simulink model "ACR_4_Saturation_5"  (R2020a)
settings: Solver=ode45  StartTime=0.0  StopTime=10.0  MaxStep=1e-5  RelTol=1e-3
libraries: simulink x1
settings Model: Creator=78253  LastModifiedBy=78253

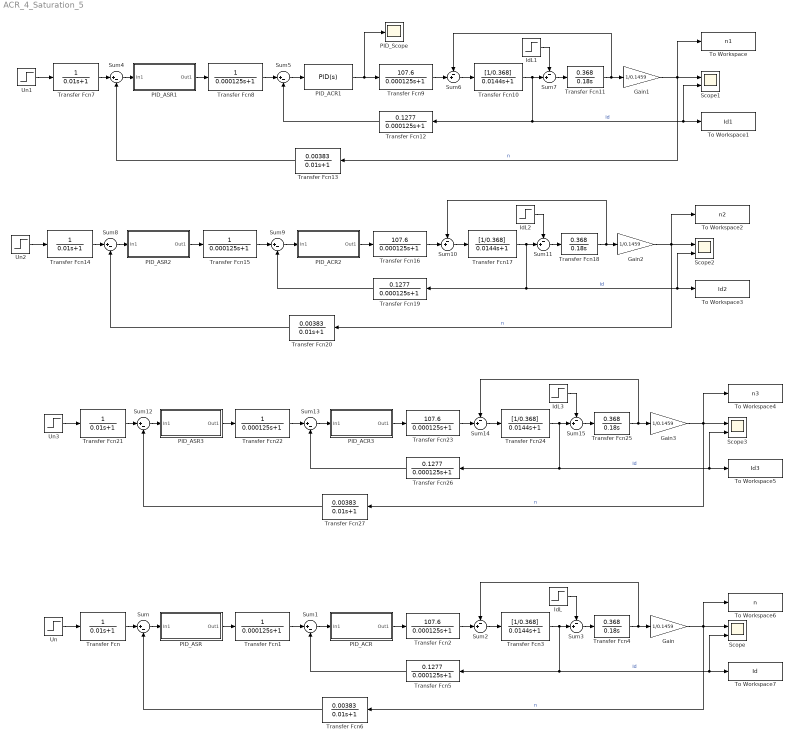
== system ACR_4_Saturation_5 ==
  Gain{,1..3} (4 alike) : Gain  Gain=1/0.1459
  IdL{,1..3} (4 alike) : Step  Time=0  After=52.2  SampleTime=0
  PID_ACR : Subsystem
  PID_ACR1 : simulink/Continuous/PID Controller  Controller=PID  Form=Parallel  TimeDomain=Continuous-time  UseExternalTs=off  SampleTime=-1  IntegratorMethod=Forward Euler  FilterMethod=Forward Euler  ControllerParametersSource=internal  P=0.771  I=53.542  D=0  UseFilter=on  N=100  TunerSelectOption=Transfer Function Based (PID Tuner App)  InitialConditionSource=internal  InitialConditionForIntegrator=0  InitialConditionForFilter=0  DifferentiatorICPrevScaledInput=0  ExternalReset=none  TrackingMode=off  Kt=1  LimitOutput=on  UpperSaturationLimit=5  LowerSaturationLimit=-5  LinearizeAsGain=on  AntiWindupMode=none  Kb=1  POutMin=[]  POutMax=[]  IOutMin=[]  IOutMax=[]  DOutMin=[]  DOutMax=[]  NOutMin=[]  NOutMax=[]  SumOutMin=[]  SumOutMax=[]  SaturationOutMin=[]  SaturationOutMax=[]  PParamMin=[]  PParamMax=[]  IParamMin=[]  IParamMax=[]  DParamMin=[]  DParamMax=[]  NParamMin=[]  NParamMax=[]  KbParamMin=[]  KbParamMax=[]  KtParamMin=[]  KtParamMax=[]  KbOutMin=[]  KbOutMax=[]  KtOutMin=[]  KtOutMax=[]  IntegratorOutMin=[]  IntegratorOutMax=[]  FilterOutMin=[]  FilterOutMax=[]  SumI1OutMin=[]  SumI1OutMax=[]  SumI2OutMin=[]  SumI2OutMax=[]  SumI3OutMin=[]  SumI3OutMax=[]  SumI4OutMin=[]  SumI4OutMax=[]  SumDOutMin=[]  SumDOutMax=[]  DifferentiatorOutMin=[]  DifferentiatorOutMax=[]  FilterDiffOutCoefMin=[]  FilterDiffOutCoefMax=[]  ReciprocalOutMin=[]  ReciprocalOutMax=[]  SumDenOutMin=[]  SumDenOutMax=[]  SumNumOutMin=[]  SumNumOutMax=[]  DivideOutMin=[]  DivideOutMax=[]  UdiffTsProdOutMin=[]  UdiffTsProdOutMax=[]  NTsProdOutMin=[]  NTsProdOutMax=[]  UintegralTsProdOutMin=[]  UintegralTsProdOutMax=[]  UngainTsProdOutMin=[]  UngainTsProdOutMax=[]  IntegratorContinuousStateAttributes=''  IntegratorStateMustResolveToSignalObject=off  IntegratorRTWStateStorageClass=Auto  FilterContinuousStateAttributes=''  FilterStateMustResolveToSignalObject=off  FilterRTWStateStorageClass=Auto  ParallelPVariant=InternalParameters  IdealPVariant=Disabled  IVariant=InternalParameters  DVariant=InternalParameters  IntegratorVariant=Continuous  SatVariant=Enabled  AWVariant=Passthrough  PCopyVariant=Disabled  TRVariant=Disabled  FdbkBlocksVariant=Forward  IdealPFdbkVariant=Disabled  SatFdbkVariant=Disabled  DerivativeFilterVariant=ContFilter  NVariant=InternalParameters  NCopyVariant=Disabled  FilterICVariant=InternalICsFilter  IntegratorICVariant=InternalICs  ExternalResetVariant=Disabled  TRSumVariant=Passthrough  SumFdbkVariant=Disabled  SumVariant=Sum_PID  TsampFilterVariant=InternalTs  TsampNgainVariant=Passthrough  TsampIntegralVariant=Passthrough
  PID_ACR2 : Subsystem
  PID_ACR3 : Subsystem
  PID_ASR : Subsystem
  PID_ASR1 : Subsystem
  PID_ASR2 : Subsystem
  PID_ASR3 : Subsystem
  PID_Scope : Scope
  Scope{,1..3} (4 alike) : Scope  NumInputPorts=2
  Sum{,1,4..5,8..9,12..13} (8 alike) : Sum  Inputs=|+-
  Sum{2..3,6..7,10..11,14..15} (8 alike) : Sum  Inputs=-+|
  To Workspace : ToWorkspace  VariableName=n1  SaveFormat=Timeseries  SampleTime=-1
  To Workspace1 : ToWorkspace  VariableName=Id1  SaveFormat=Timeseries  SampleTime=-1
  To Workspace2 : ToWorkspace  VariableName=n2  SaveFormat=Timeseries  SampleTime=-1
  To Workspace3 : ToWorkspace  VariableName=Id2  SaveFormat=Timeseries  SampleTime=-1
  To Workspace4 : ToWorkspace  VariableName=n3  SaveFormat=Timeseries  SampleTime=-1
  To Workspace5 : ToWorkspace  VariableName=Id3  SaveFormat=Timeseries  SampleTime=-1
  To Workspace6 : ToWorkspace  VariableName=n  SaveFormat=Timeseries  SampleTime=-1
  To Workspace7 : ToWorkspace  VariableName=Id  SaveFormat=Timeseries  SampleTime=-1
  Transfer Fcn{,7,14,21} (4 alike) : TransferFcn  Denominator=[0.01 1]
  Transfer Fcn{1,8,15,22} (4 alike) : TransferFcn  Denominator=[0.000125 1]
  Transfer Fcn{3,10,17,24} (4 alike) : TransferFcn  Numerator=[1/0.368]  Denominator=[0.0144 1]
  Transfer Fcn{4,11,18,25} (4 alike) : TransferFcn  Numerator=[0.368]  Denominator=[0.18 0]
  Transfer Fcn{5,12,19,26} (4 alike) : TransferFcn  Numerator=[0.1277]  Denominator=[0.000125 1]
  Transfer Fcn{6,13,20,27} (4 alike) : TransferFcn  Numerator=[0.00383]  Denominator=[0.01 1]
  Transfer Fcn{2,9,16,23} (4 alike) : TransferFcn  Numerator=[107.6]  Denominator=[0.000125 1]
  Un{,1..3} (4 alike) : Step  Time=0  After=10  SampleTime=0
  wires:
  Sum3/1 -> Transfer Fcn4/1
  Transfer Fcn/1 -> Sum/1
  Sum2/1 -> Transfer Fcn3/1
  Un/1 -> Transfer Fcn/1
  Transfer Fcn5/1 -> Sum1/2
  Transfer Fcn6/1 -> Sum/2
  PID_ACR/1(Out1) -> Transfer Fcn2/1
  Transfer Fcn1/1 -> Sum1/1
  IdL/1 -> Sum3/1
  Transfer Fcn4/1 -> Sum2/1, Gain/1
  Transfer Fcn3/1 -> Transfer Fcn5/1, Scope/2, To Workspace7/1, Sum3/2  "Id"
  Gain/1 -> To Workspace6/1, Transfer Fcn6/1, Scope/1  "n"
  Sum/1 -> PID_ASR/1(In1)
  Sum1/1 -> PID_ACR/1(In1)
  Transfer Fcn2/1 -> Sum2/2
  PID_ASR/1(Out1) -> Transfer Fcn1/1
  PID_ASR1/1(Out1) -> Transfer Fcn8/1
  Transfer Fcn10/1 -> Transfer Fcn12/1, Scope1/2, To Workspace1/1, Sum7/2  "Id"
  Transfer Fcn9/1 -> Sum6/2
  Gain1/1 -> To Workspace/1, Transfer Fcn13/1, Scope1/1  "n"
  Transfer Fcn8/1 -> Sum5/1
  Transfer Fcn13/1 -> Sum4/2
  Sum4/1 -> PID_ASR1/1(In1)
  IdL1/1 -> Sum7/1
  Transfer Fcn7/1 -> Sum4/1
  Transfer Fcn12/1 -> Sum5/2
  Un1/1 -> Transfer Fcn7/1
  Sum6/1 -> Transfer Fcn10/1
  Transfer Fcn11/1 -> Sum6/1, Gain1/1
  Sum7/1 -> Transfer Fcn11/1
  PID_ASR2/1(Out1) -> Transfer Fcn15/1
  Transfer Fcn17/1 -> Transfer Fcn19/1, To Workspace3/1, Scope2/2, Sum11/2  "Id"
  Transfer Fcn16/1 -> Sum10/2
  Gain2/1 -> To Workspace2/1, Transfer Fcn20/1, Scope2/1  "n"
  Sum9/1 -> PID_ACR2/1(In1)
  Transfer Fcn15/1 -> Sum9/1
  Transfer Fcn20/1 -> Sum8/2
  PID_ACR2/1(Out1) -> Transfer Fcn16/1
  Sum8/1 -> PID_ASR2/1(In1)
  IdL2/1 -> Sum11/1
  Transfer Fcn14/1 -> Sum8/1
  Transfer Fcn19/1 -> Sum9/2
  Un2/1 -> Transfer Fcn14/1
  Sum10/1 -> Transfer Fcn17/1
  Transfer Fcn18/1 -> Sum10/1, Gain2/1
  Sum11/1 -> Transfer Fcn18/1
  PID_ASR3/1(Out1) -> Transfer Fcn22/1
  Transfer Fcn24/1 -> Transfer Fcn26/1, To Workspace5/1, Scope3/2, Sum15/2  "Id"
  Transfer Fcn23/1 -> Sum14/2
  Gain3/1 -> To Workspace4/1, Transfer Fcn27/1, Scope3/1  "n"
  Sum13/1 -> PID_ACR3/1(In1)
  Transfer Fcn22/1 -> Sum13/1
  Transfer Fcn27/1 -> Sum12/2
  PID_ACR3/1(Out1) -> Transfer Fcn23/1
  Sum12/1 -> PID_ASR3/1(In1)
  IdL3/1 -> Sum15/1
  Transfer Fcn21/1 -> Sum12/1
  Transfer Fcn26/1 -> Sum13/2
  Un3/1 -> Transfer Fcn21/1
  Sum14/1 -> Transfer Fcn24/1
  Transfer Fcn25/1 -> Sum14/1, Gain3/1
  Sum15/1 -> Transfer Fcn25/1
  PID_ACR1/1 -> PID_Scope/1, Transfer Fcn9/1
  Sum5/1 -> PID_ACR1/1

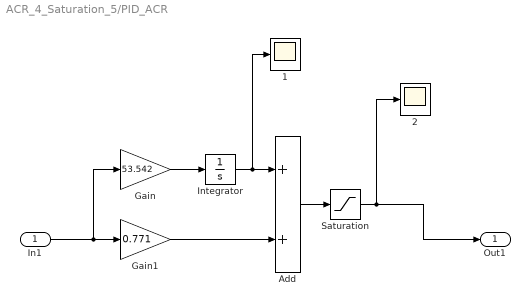
== system ACR_4_Saturation_5/PID_ACR ==
  In1 : Inport
  1 : Scope
  2 : Scope
  Add : Sum
  Gain : Gain  Gain=53.542
  Gain1 : Gain  Gain=0.771
  Integrator : Integrator  LimitOutput=on  UpperSaturationLimit=5  LowerSaturationLimit=-5
  Saturation : Saturate  UpperLimit=5  LowerLimit=-5
  Out1 : Outport
  wires:
  In1/1 -> Gain/1, Gain1/1
  Gain1/1 -> Add/2
  Add/1 -> Saturation/1
  Gain/1 -> Integrator/1
  Saturation/1 -> Out1/1, 2/1
  Integrator/1 -> 1/1, Add/1

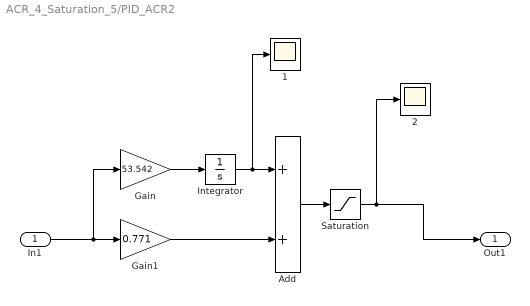
== system ACR_4_Saturation_5/PID_ACR2 ==
  In1 : Inport
  1 : Scope
  2 : Scope
  Add : Sum
  Gain : Gain  Gain=53.542
  Gain1 : Gain  Gain=0.771
  Integrator : Integrator  UpperSaturationLimit=5  LowerSaturationLimit=-5
  Saturation : Saturate  UpperLimit=5  LowerLimit=-5
  Out1 : Outport
  wires:
  In1/1 -> Gain/1, Gain1/1
  Gain1/1 -> Add/2
  Add/1 -> Saturation/1
  Gain/1 -> Integrator/1
  Saturation/1 -> Out1/1, 2/1
  Integrator/1 -> 1/1, Add/1

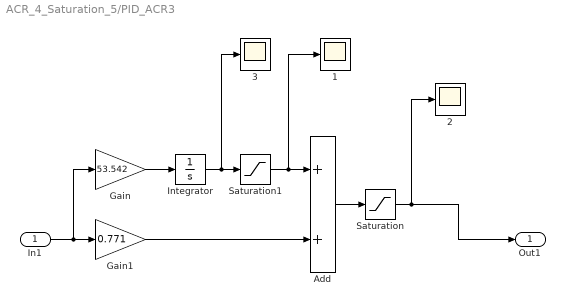
== system ACR_4_Saturation_5/PID_ACR3 ==
  In1 : Inport
  1 : Scope
  2 : Scope
  3 : Scope
  Add : Sum
  Gain : Gain  Gain=53.542
  Gain1 : Gain  Gain=0.771
  Integrator : Integrator  UpperSaturationLimit=5  LowerSaturationLimit=-5
  Saturation : Saturate  UpperLimit=5  LowerLimit=-5
  Saturation1 : Saturate  UpperLimit=5  LowerLimit=-5
  Out1 : Outport
  wires:
  In1/1 -> Gain1/1, Gain/1
  Gain1/1 -> Add/2
  Add/1 -> Saturation/1
  Gain/1 -> Integrator/1
  Saturation/1 -> Out1/1, 2/1
  Integrator/1 -> 3/1, Saturation1/1
  Saturation1/1 -> 1/1, Add/1

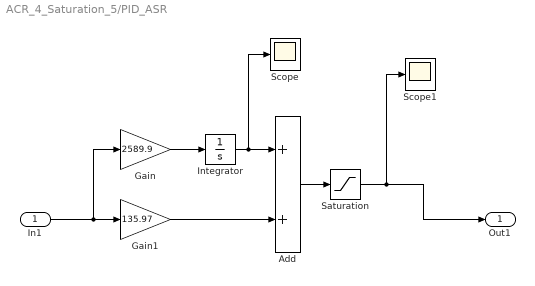
== system ACR_4_Saturation_5/PID_ASR ==
  In1 : Inport
  Add : Sum
  Gain : Gain  Gain=2589.9
  Gain1 : Gain  Gain=135.97
  Integrator : Integrator  LimitOutput=on  UpperSaturationLimit=10  LowerSaturationLimit=-10
  Saturation : Saturate  UpperLimit=10  LowerLimit=-10
  Scope : Scope
  Scope1 : Scope
  Out1 : Outport
  wires:
  In1/1 -> Gain/1, Gain1/1
  Gain/1 -> Integrator/1
  Gain1/1 -> Add/2
  Integrator/1 -> Scope/1, Add/1
  Add/1 -> Saturation/1
  Saturation/1 -> Scope1/1, Out1/1

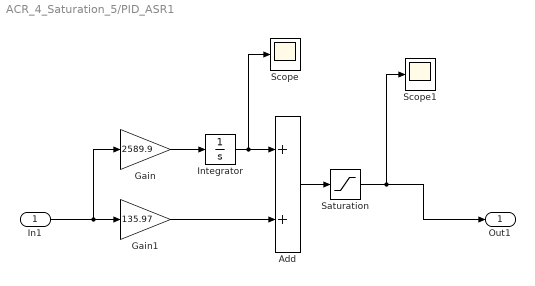
== system ACR_4_Saturation_5/PID_ASR1 ==
  In1 : Inport
  Add : Sum
  Gain : Gain  Gain=2589.9
  Gain1 : Gain  Gain=135.97
  Integrator : Integrator  LimitOutput=on  UpperSaturationLimit=10  LowerSaturationLimit=-10
  Saturation : Saturate  UpperLimit=10  LowerLimit=-10
  Scope : Scope
  Scope1 : Scope
  Out1 : Outport
  wires:
  In1/1 -> Gain/1, Gain1/1
  Gain/1 -> Integrator/1
  Gain1/1 -> Add/2
  Integrator/1 -> Scope/1, Add/1
  Add/1 -> Saturation/1
  Saturation/1 -> Scope1/1, Out1/1

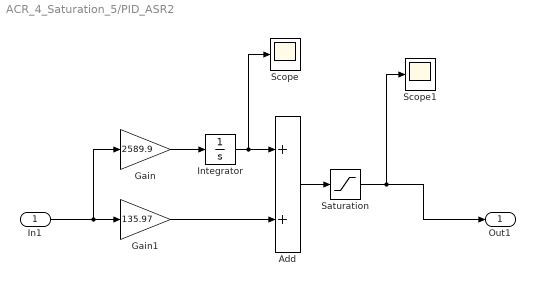
== system ACR_4_Saturation_5/PID_ASR2 ==
  In1 : Inport
  Add : Sum
  Gain : Gain  Gain=2589.9
  Gain1 : Gain  Gain=135.97
  Integrator : Integrator  LimitOutput=on  UpperSaturationLimit=10  LowerSaturationLimit=-10
  Saturation : Saturate  UpperLimit=10  LowerLimit=-10
  Scope : Scope
  Scope1 : Scope
  Out1 : Outport
  wires:
  In1/1 -> Gain/1, Gain1/1
  Gain/1 -> Integrator/1
  Gain1/1 -> Add/2
  Integrator/1 -> Scope/1, Add/1
  Add/1 -> Saturation/1
  Saturation/1 -> Scope1/1, Out1/1

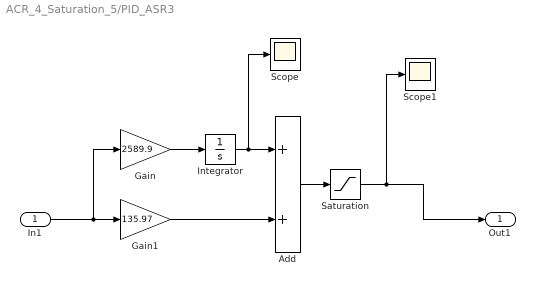
== system ACR_4_Saturation_5/PID_ASR3 ==
  In1 : Inport
  Add : Sum
  Gain : Gain  Gain=2589.9
  Gain1 : Gain  Gain=135.97
  Integrator : Integrator  LimitOutput=on  UpperSaturationLimit=10  LowerSaturationLimit=-10
  Saturation : Saturate  UpperLimit=10  LowerLimit=-10
  Scope : Scope
  Scope1 : Scope
  Out1 : Outport
  wires:
  In1/1 -> Gain/1, Gain1/1
  Gain/1 -> Integrator/1
  Gain1/1 -> Add/2
  Integrator/1 -> Scope/1, Add/1
  Add/1 -> Saturation/1
  Saturation/1 -> Scope1/1, Out1/1
